simulink model "LotkaVolterra"  (R2024b)
settings: Solver=ode4  StartTime=0.0  StopTime=50.0  FixedStep=0.01  RelTol=1e-3
model workspace (MATLAB code in the model file):
  | alpha = 1;
  | beta = 1;
  | gamma = 1;
  | delta = 1;
settings Model: Creator=Miguel  LastModifiedBy=Miguel

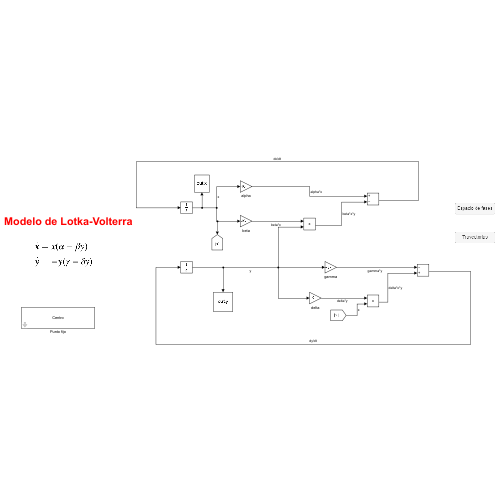
[thumbnail: Simulink's stored preview of the top-level diagram]
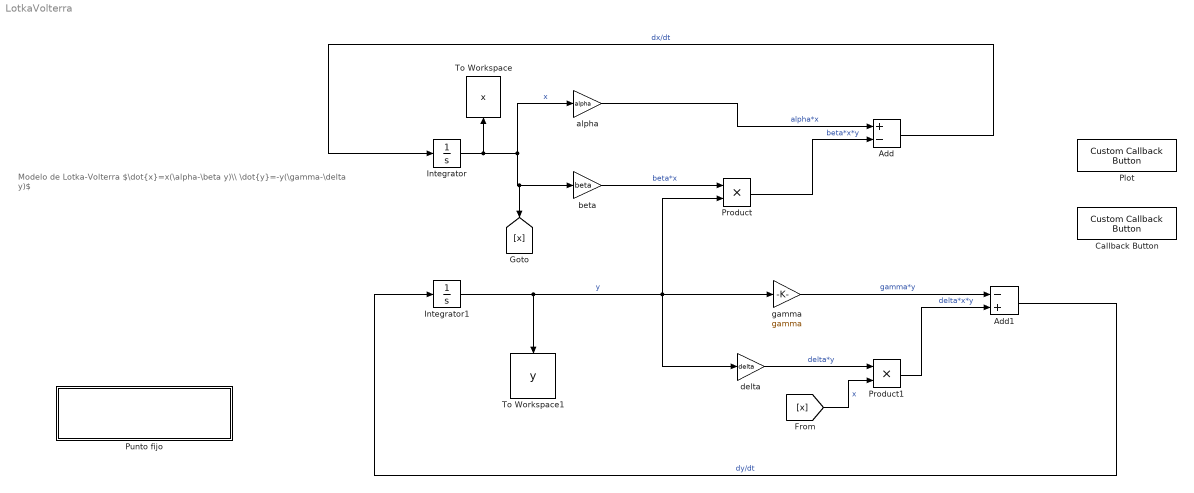
== system LotkaVolterra ==
  note: Modelo de Lotka-Volterra
      |
      | $\dot{x}=x(\alpha-\beta y)\\ \dot{y}=-y(\gamma-\delta y)$
  Add : Sum  Inputs=+-
  Add1 : Sum  Inputs=-+
  Callback Button : CustomCallbackButton  Configuration="{\"components\":[{\"name\":\"BackgroundImageComponent\",\"settings\":{\"image\":{\"size\":[0,0],\"src\":\"default\",\"srcOrientation\":\"Right\"},\"position\":[0,0,1,1]}},{\"name\":\"ButtonStateComponent\",\"settings\":{\"buttonType\":\"momentary\",\"clickFcn\":\"x = out.x;\\ny = out.y;\\nt = out.tout;\\n\\nfigure\\nplot(t, x, 'linewidth', 2)\\nhold on\\ngrid on\\nplot(t, y, 'linewidth', 2)\\nxlabel('Tiempo')\\nylabel('Población')\\nlegend('x', 'y')\\ntitle('Trayectorias')\",\"onValue\":1,\"position\":[0,0,1,1],\"pressDelay\":\"500\",\"pressFcn\":\"\",\"repeatInterval\":\"0\",\"states\":[{\"horizontalAlignment\":\"center\",\"image\":{\"position\":[0,0,1,1],\"size\":[1,1],\"src\":\"default\",\"srcOrientation\":\"Right\"},\"label\":{\"color\":[0.01176470588,0.01176470588,0.01176470588,1],\"icon\":{\"size\":[0,0],\"src\":\"default\",\"srcOrientation\":\"Right\"},\"iconOffset\":0,\"iconPlacement\":\"left\",\"opacity\":1,\"show\":true,\"text\":{\"content\":\"Trayectorias\",\"font\":\"Helvetica\"}},\"labelOffset\":[0,0],\"verticalAlignment\":\"middle\"},{\"horizontalAlignment\":\"center\",\"image\":{\"position\":[0,0,1,1],\"size\":[1,1],\"src\":\"default\",\"srcOrientation\":\"Right\"},\"label\":{\"color\":[0.01176470588,0.01176470588,0.01176470588,1],\"icon\":{\"size\":[0,0],\"src\":\"default\",\"srcOrientation\":\"Right\"},\"iconOffset\":0,\"iconPlacement\":\"left\",\"opacity\":1,\"show\":true,\"text\":{\"content\":\"Trayectorias\",\"font\":\"Helvetica\"}},\"labelOffset\":[0,0],\"verticalAlignment\":\"middle\"},{\"horizontalAlignment\":\"center\",\"image\":{\"position\":[0,0,1,1],\"size\":[1,1],\"src\":\"default\",\"srcOrientation\":\"Right\"},\"label\":{\"color\":[0.01176470588,0.01176470588,0.01176470588,1],\"icon\":{\"size\":[0,0],\"src\":\"default\",\"srcOrientation\":\"Right\"},\"iconOffset\":0,\"iconPlacement\":\"left\",\"opacity\":1,\"show\":true,\"text\":{\"content\":\"Trayectorias\",\"font\":\"Helvetica\"}},\"labelOffset\":[0,0],\"verticalAlignment\":\"middle\"},{\"horizontalAlignment\":\"center\",\"image\":{\"position\":[0,0,1,1],\"size\":[1,1],\"src\":\"default\",\"srcOrientation\":\"Right\"},\"label\":{\"color\":[0.01176470588,0.01176470588,0.01176470588,1],\"icon\":{\"size\":[0,0],\"src\":\"default\",\"srcOrientation\":\"Right\"},\"iconOffset\":0,\"iconPlacement\":\"left\",\"opacity\":1,\"show\":true,\"text\":{\"content\":\"Trayectorias\",\"font\":\"Helvetica\"}},\"labelOffset\":[0,0],\"verticalAlignment\":\"middle\"}]}},{\"name\":\"ForegroundImageComponent\",\"settings\":{\"image\":{\"size\":[0,0],\"src\":\"default\",\"srcOrientation\":\"Right\"},\"isForeground\":1,\"position\":[0,0,1,1]}}],\"settings\":{\"BindingType\":\"standalone\",\"backgroundColor\":[244,244,244,1],\"backgroundOffset\":0.2,\"backgroundOpacity\":1,\"fixedAspectRatio\":\"off\",\"foregroundColor\":[0.01176470588,0.01176470588,0.01176470588,1],\"migratedFromLegacy\":true,\"useBackgroundColor\":true,\"variant\":\"callback\",\"version\":\"R2023a\"},\"type\":\"Button\"}"  CustomBackgroundColor="{\"color\":[0.9568627451,0.9568627451,0.9568627451],\"show\":true}"
  Integrator : Integrator  InitialCondition=linspace(0,2,10)
  Integrator1 : Integrator  InitialCondition=0.2
  Plot : CustomCallbackButton  Configuration="{\"components\":[{\"name\":\"BackgroundImageComponent\",\"settings\":{\"image\":{\"size\":[0,0],\"src\":\"default\",\"srcOrientation\":\"Right\"},\"position\":[0,0,1,1]}},{\"name\":\"ButtonStateComponent\",\"settings\":{\"buttonType\":\"momentary\",\"clickFcn\":\"x = out.x;\\ny = out.y;\\nx_centro = out.x_centro;\\ny_centro = out.y_centro;\\n\\n% Trayectorias en el espacio de fases\\nfigure\\nplot(x, y, 'linewidth', 2)\\nhold on\\n\\n% Ubicación del punto fijo centro\\nplot(x_centro, y_centro, 'ro', 'MarkerEdgeColor', 'r', 'MarkerFaceColor', 'r', 'MarkerSize', 6)\\n\\ngrid on\\nxlabel('x')\\nylabel('y')\\ntitle('Espacio de fases')\",\"onValue\":1,\"position\":[0,0,1,1],\"pressDelay\":\"500\",\"pressFcn\":\"\",\"repeatInterval\":\"0\",\"states\":[{\"horizontalAlignment\":\"center\",\"image\":{\"position\":[0,0,1,1],\"size\":[1,1],\"src\":\"default\",\"srcOrientation\":\"Right\"},\"label\":{\"color\":[0.01176470588,0.01176470588,0.01176470588,1],\"icon\":{\"size\":[0,0],\"src\":\"default\",\"srcOrientation\":\"Right\"},\"iconOffset\":0,\"iconPlacement\":\"left\",\"opacity\":1,\"show\":true,\"text\":{\"content\":\"Espacio de fases\",\"font\":\"Helvetica\"}},\"labelOffset\":[0,0],\"verticalAlignment\":\"middle\"},{\"horizontalAlignment\":\"center\",\"image\":{\"position\":[0,0,1,1],\"size\":[1,1],\"src\":\"default\",\"srcOrientation\":\"Right\"},\"label\":{\"color\":[0.01176470588,0.01176470588,0.01176470588,1],\"icon\":{\"size\":[0,0],\"src\":\"default\",\"srcOrientation\":\"Right\"},\"iconOffset\":0,\"iconPlacement\":\"left\",\"opacity\":1,\"show\":true,\"text\":{\"content\":\"Espacio de fases\",\"font\":\"Helvetica\"}},\"labelOffset\":[0,0],\"verticalAlignment\":\"middle\"},{\"horizontalAlignment\":\"center\",\"image\":{\"position\":[0,0,1,1],\"size\":[1,1],\"src\":\"default\",\"srcOrientation\":\"Right\"},\"label\":{\"color\":[0.01176470588,0.01176470588,0.01176470588,1],\"icon\":{\"size\":[0,0],\"src\":\"default\",\"srcOrientation\":\"Right\"},\"iconOffset\":0,\"iconPlacement\":\"left\",\"opacity\":1,\"show\":true,\"text\":{\"content\":\"Espacio de fases\",\"font\":\"Helvetica\"}},\"labelOffset\":[0,0],\"verticalAlignment\":\"middle\"},{\"horizontalAlignment\":\"center\",\"image\":{\"position\":[0,0,1,1],\"size\":[1,1],\"src\":\"default\",\"srcOrientation\":\"Right\"},\"label\":{\"color\":[0.01176470588,0.01176470588,0.01176470588,1],\"icon\":{\"size\":[0,0],\"src\":\"default\",\"srcOrientation\":\"Right\"},\"iconOffset\":0,\"iconPlacement\":\"left\",\"opacity\":1,\"show\":true,\"text\":{\"content\":\"Espacio de fases\",\"font\":\"Helvetica\"}},\"labelOffset\":[0,0],\"verticalAlignment\":\"middle\"}]}},{\"name\":\"ForegroundImageComponent\",\"settings\":{\"image\":{\"size\":[0,0],\"src\":\"default\",\"srcOrientation\":\"Right\"},\"isForeground\":1,\"position\":[0,0,1,1]}}],\"settings\":{\"BindingType\":\"standalone\",\"backgroundColor\":[244,244,244,1],\"backgroundOffset\":0.2,\"backgroundOpacity\":1,\"fixedAspectRatio\":\"off\",\"foregroundColor\":[0.01176470588,0.01176470588,0.01176470588,1],\"migratedFromLegacy\":true,\"useBackgroundColor\":true,\"variant\":\"callback\",\"version\":\"R2023a\"},\"type\":\"Button\"}"  CustomBackgroundColor="{\"color\":[0.9568627451,0.9568627451,0.9568627451],\"show\":true}"
  Product : Product
  Product1 : Product
  Punto fijo : Subsystem
      mask Display: disp('Centro')
  To Workspace : ToWorkspace  VariableName=x  SampleTime=-1
  To Workspace1 : ToWorkspace  VariableName=y  SampleTime=-1
  alpha : Gain  Gain=alpha
  beta : Gain  Gain=beta
  delta : Gain  Gain=delta
  gamma : Gain  Gain=gamma
  wires:
  Integrator/1 -> alpha/1, [x], beta/1, To Workspace/1  "x"
  alpha/1 -> Add/1  "alpha*x"
  beta/1 -> Product/1  "beta*x"
  Integrator1/1 -> To Workspace1/1, delta/1, gamma/1, Product/2  "y"
  Product/1 -> Add/2  "beta*x*y"
  Add/1 -> Integrator/1  "dx/dt"
  delta/1 -> Product1/1  "delta*y"
  [x] -> Product1/2  "x"
  gamma/1 -> Add1/1  "gamma*y"
  Product1/1 -> Add1/2  "delta*x*y"
  Add1/1 -> Integrator1/1  "dy/dt"

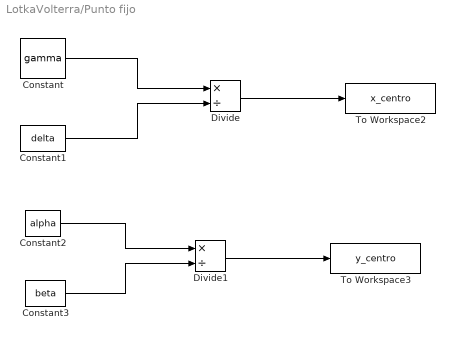
== system LotkaVolterra/Punto fijo ==
  Constant : Constant  Value=gamma
  Constant1 : Constant  Value=delta
  Constant2 : Constant  Value=alpha
  Constant3 : Constant  Value=beta
  Divide : Product  Inputs=*/
  Divide1 : Product  Inputs=*/
  To Workspace2 : ToWorkspace  VariableName=x_centro  SampleTime=-1
  To Workspace3 : ToWorkspace  VariableName=y_centro  SampleTime=-1
  wires:
  Constant2/1 -> Divide1/1
  Divide1/1 -> To Workspace3/1
  Constant/1 -> Divide/1
  Divide/1 -> To Workspace2/1
  Constant1/1 -> Divide/2
  Constant3/1 -> Divide1/2
